simulink model "Ej6_7_showcase_model"  (R2018a)
settings: Solver=VariableStepAuto  StartTime=0.0  StopTime=200  RelTol=1e-3
libraries: simulink x1
settings Model: Creator=joses  LastModifiedBy=joses

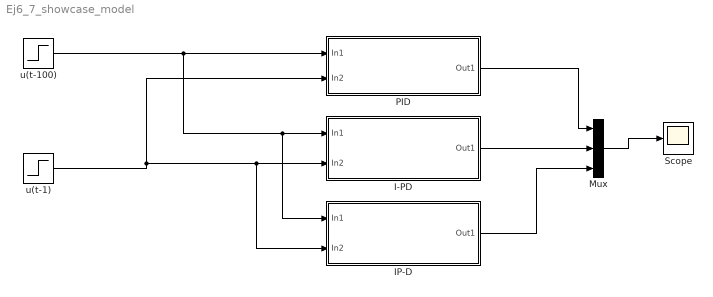
== system Ej6_7_showcase_model ==
  I-PD : Subsystem
  IP-D : Subsystem
  Mux : Mux  Inputs=3
  PID : Subsystem
  Scope : Scope
  u(t-1) : Step  SampleTime=0
  u(t-100) : Step  Time=100  SampleTime=0
  wires:
  u(t-1)/1 -> PID/2(In2), IP-D/2(In2), I-PD/2(In2)
  u(t-100)/1 -> IP-D/1(In1), I-PD/1(In1), PID/1(In1)
  Mux/1 -> Scope/1
  I-PD/1(Out1) -> Mux/2
  PID/1(Out1) -> Mux/1
  IP-D/1(Out1) -> Mux/3

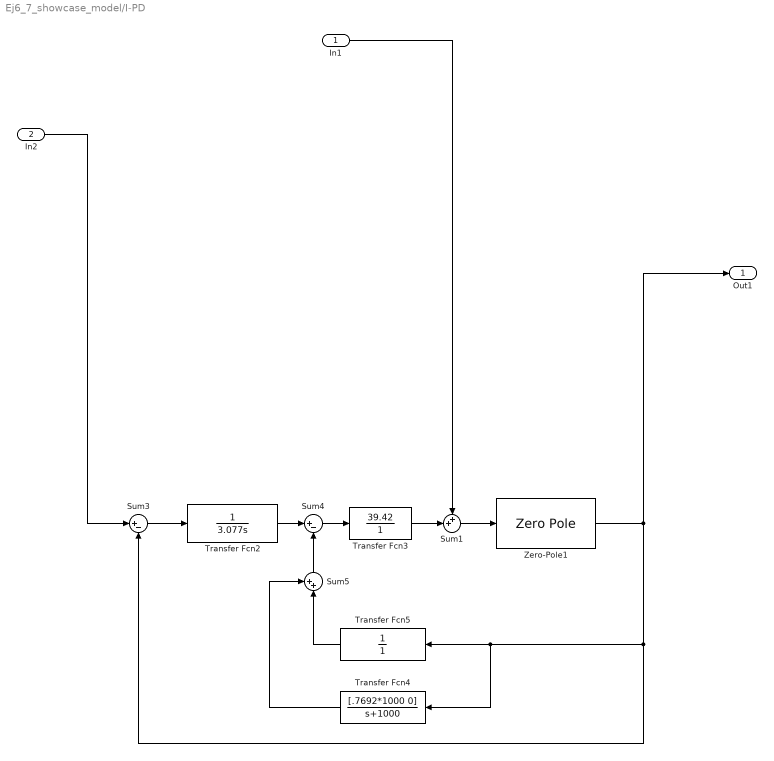
== system Ej6_7_showcase_model/I-PD ==
  In1 : Inport
  In2 : Inport  Port=2
  Sum1 : Sum  Inputs=++|
  Sum3 : Sum  Inputs=|+-
  Sum4 : Sum  Inputs=|+-
  Sum5 : Sum  Inputs=++|
  Transfer Fcn2 : TransferFcn  Denominator=[3.077 0]
  Transfer Fcn3 : TransferFcn  Numerator=[39.42]  Denominator=[1]
  Transfer Fcn4 : TransferFcn  Numerator=[.7692*1000 0]  Denominator=[1 1000]
  Transfer Fcn5 : TransferFcn  Numerator=1  Denominator=1
  Zero-Pole1 : ZeroPole  Zeros=[]  Poles=[0 -1 -5]
  Out1 : Outport
  wires:
  Transfer Fcn3/1 -> Sum1/2
  Transfer Fcn5/1 -> Sum5/2
  Sum4/1 -> Transfer Fcn3/1
  Zero-Pole1/1 -> Out1/1, Transfer Fcn5/1, Transfer Fcn4/1, Sum3/2
  Transfer Fcn2/1 -> Sum4/1
  In1/1 -> Sum1/1
  Sum1/1 -> Zero-Pole1/1
  Sum5/1 -> Sum4/2
  Transfer Fcn4/1 -> Sum5/1
  Sum3/1 -> Transfer Fcn2/1
  In2/1 -> Sum3/1

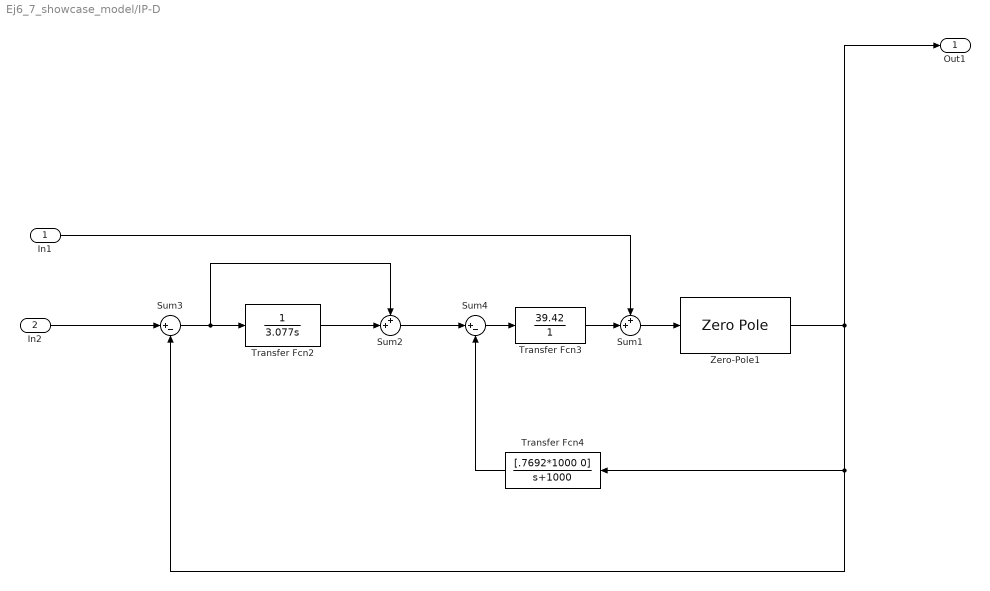
== system Ej6_7_showcase_model/IP-D ==
  In1 : Inport
  In2 : Inport  Port=2
  Sum1 : Sum  Inputs=++|
  Sum2 : Sum  Inputs=++|
  Sum3 : Sum  Inputs=|+-
  Sum4 : Sum  Inputs=|+-
  Transfer Fcn2 : TransferFcn  Denominator=[3.077 0]
  Transfer Fcn3 : TransferFcn  Numerator=[39.42]  Denominator=[1]
  Transfer Fcn4 : TransferFcn  Numerator=[.7692*1000 0]  Denominator=[1 1000]
  Zero-Pole1 : ZeroPole  Zeros=[]  Poles=[0 -1 -5]
  Out1 : Outport
  wires:
  Transfer Fcn3/1 -> Sum1/2
  Zero-Pole1/1 -> Out1/1, Sum3/2, Transfer Fcn4/1
  Sum4/1 -> Transfer Fcn3/1
  In1/1 -> Sum1/1
  Sum1/1 -> Zero-Pole1/1
  Transfer Fcn4/1 -> Sum4/2
  In2/1 -> Sum3/1
  Sum3/1 -> Sum2/1, Transfer Fcn2/1
  Transfer Fcn2/1 -> Sum2/2
  Sum2/1 -> Sum4/1

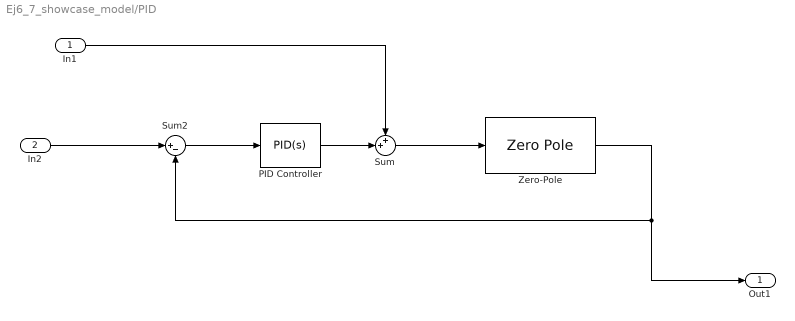
== system Ej6_7_showcase_model/PID ==
  In1 : Inport
  In2 : Inport  Port=2
  PID Controller : simulink/Continuous/PID Controller  Controller=PID  TimeDomain=Continuous-time  SampleTime=-1  IntegratorMethod=Forward Euler  FilterMethod=Forward Euler  Form=Ideal  UseFilter=on  ControllerParametersSource=internal  P=39.42  I=1/3.077  D=.7692  N=100  InitialConditionSource=internal  InitialConditionForIntegrator=0  InitialConditionForFilter=0  ExternalReset=none  LimitOutput=off  UpperSaturationLimit=inf  LowerSaturationLimit=-inf  LinearizeAsGain=on  AntiWindupMode=none  Kb=1  TrackingMode=off  Kt=1  PParamMin=[]  PParamMax=[]  IParamMin=[]  IParamMax=[]  DParamMin=[]  DParamMax=[]  NParamMin=[]  NParamMax=[]  KbParamMin=[]  KbParamMax=[]  KtParamMin=[]  KtParamMax=[]  POutMin=[]  POutMax=[]  IOutMin=[]  IOutMax=[]  DOutMin=[]  DOutMax=[]  NOutMin=[]  NOutMax=[]  KbOutMin=[]  KbOutMax=[]  KtOutMin=[]  KtOutMax=[]  IntegratorOutMin=[]  IntegratorOutMax=[]  FilterOutMin=[]  FilterOutMax=[]  SumOutMin=[]  SumOutMax=[]  SumI1OutMin=[]  SumI1OutMax=[]  SumI2OutMin=[]  SumI2OutMax=[]  SumI3OutMin=[]  SumI3OutMax=[]  SumDOutMin=[]  SumDOutMax=[]  SaturationOutMin=[]  SaturationOutMax=[]  IntegratorContinuousStateAttributes=''  IntegratorStateMustResolveToSignalObject=off  IntegratorRTWStateStorageClass=Auto  FilterContinuousStateAttributes=''  FilterStateMustResolveToSignalObject=off  FilterRTWStateStorageClass=Auto  DifferentiatorICPrevScaledInput=0  DifferentiatorOutMin=[]  DifferentiatorOutMax=[]  FilterDiffOutCoefMin=[]  FilterDiffOutCoefMax=[]  SumDenOutMin=[]  SumDenOutMax=[]  SumNumOutMin=[]  SumNumOutMax=[]  ReciprocalOutMin=[]  ReciprocalOutMax=[]  DivideOutMin=[]  DivideOutMax=[]  TunerSelectOption=Transfer Function Based (PID Tuner App)
  Sum : Sum  Inputs=++|
  Sum2 : Sum  Inputs=|+-
  Zero-Pole : ZeroPole  Zeros=[]  Poles=[0 -1 -5]
  Out1 : Outport
  wires:
  Sum2/1 -> PID Controller/1
  In1/1 -> Sum/1
  Zero-Pole/1 -> Out1/1, Sum2/2
  Sum/1 -> Zero-Pole/1
  PID Controller/1 -> Sum/2
  In2/1 -> Sum2/1
